simulink model "OAC_LA_Ass1_Task2_simu_R2017b"  (R2017b)
settings: Solver=VariableStepAuto  StartTime=0.0  StopTime=10.0  MaxStep=10e-3  RelTol=1e-3
undefined symbols (not defined in the file): g, l, params_L1, params_L2, params_Linfty, x0
settings Model: Creator=miko2  LastModifiedBy=miko2

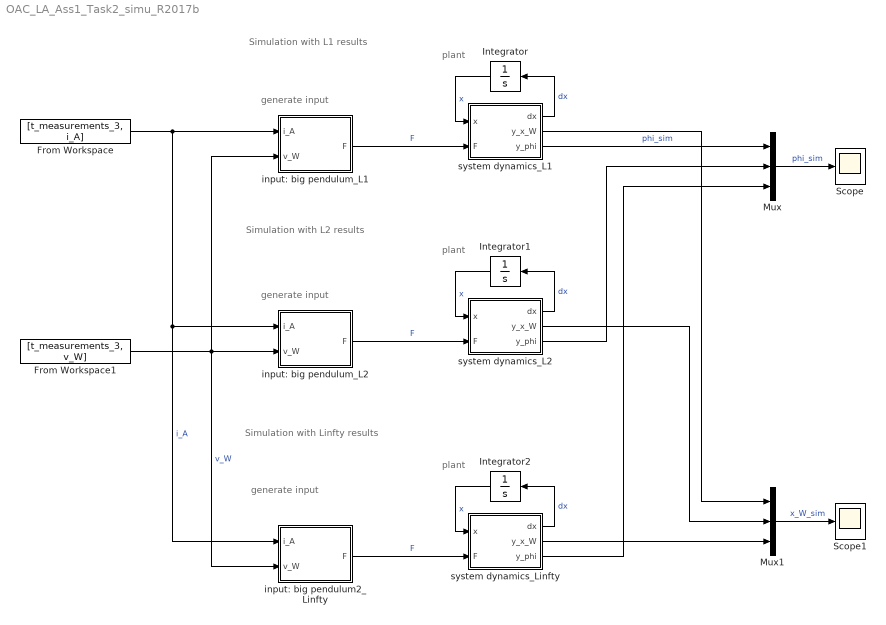
== system OAC_LA_Ass1_Task2_simu_R2017b ==
  note: Simulation with Linfty results
  note: Simulation with L2 results
  note: Simulation with L1 results
  note: generate input
  note: plant
  note: plant
  note: plant
  note: generate input
  note: generate input
  From Workspace : FromWorkspace  VariableName=[t_measurements_3, i_A]  SampleTime=0
  From Workspace1 : FromWorkspace  VariableName=[t_measurements_3, v_W]  SampleTime=0
  Integrator : Integrator  InitialCondition=x0
  Integrator1 : Integrator  InitialCondition=x0
  Integrator2 : Integrator  InitialCondition=x0
  Mux : Mux  Inputs=3
  Mux1 : Mux  Inputs=3
  Scope : Scope
  Scope1 : Scope
  input: big pendulum2_Linfty : MATLAB Function  TreatAsAtomicUnit=on
  input: big pendulum_L1 : MATLAB Function  TreatAsAtomicUnit=on
  input: big pendulum_L2 : MATLAB Function  TreatAsAtomicUnit=on
  system dynamics_L1 : MATLAB Function  TreatAsAtomicUnit=on
  system dynamics_L2 : MATLAB Function  TreatAsAtomicUnit=on
  system dynamics_Linfty : MATLAB Function  TreatAsAtomicUnit=on
  wires:
  system dynamics_L1/3(y_phi) -> Mux/1  "phi_sim"
  Integrator/1 -> system dynamics_L1/1(x)  "x"
  input: big pendulum_L1/1(F) -> system dynamics_L1/2(F)  "F"
  From Workspace/1 -> input: big pendulum_L1/1(i_A), input: big pendulum_L2/1(i_A), input: big pendulum2_Linfty/1(i_A)  "i_A"
  From Workspace1/1 -> input: big pendulum_L2/2(v_W), input: big pendulum_L1/2(v_W), input: big pendulum2_Linfty/2(v_W)  "v_W"
  system dynamics_L1/1(dx) -> Integrator/1  "dx"
  Integrator1/1 -> system dynamics_L2/1(x)  "x"
  system dynamics_L2/1(dx) -> Integrator1/1  "dx"
  system dynamics_L2/3(y_phi) -> Mux/2
  Integrator2/1 -> system dynamics_Linfty/1(x)  "x"
  system dynamics_Linfty/1(dx) -> Integrator2/1  "dx"
  system dynamics_Linfty/3(y_phi) -> Mux/3
  input: big pendulum_L2/1(F) -> system dynamics_L2/2(F)  "F"
  input: big pendulum2_Linfty/1(F) -> system dynamics_Linfty/2(F)  "F"
  Mux/1 -> Scope/1  "phi_sim"
  system dynamics_L1/2(y_x_W) -> Mux1/1
  system dynamics_L2/2(y_x_W) -> Mux1/2
  system dynamics_Linfty/2(y_x_W) -> Mux1/3
  Mux1/1 -> Scope1/1  "x_W_sim"

== matlab function OAC_LA_Ass1_Task2_simu_R2017b/input: big pendulum_L1 ==
  data: i_A input; v_W input; F output; params_L1 parameter
function F = fcn(i_A, v_W, params_L1)
    
    V = params_L1(3);
    k1 = params_L1(4);

    F = V*i_A - k1*v_W;

end

== matlab function OAC_LA_Ass1_Task2_simu_R2017b/system dynamics_L1 ==
  data: dx output; x input; y_x_W output; F input; y_phi output; params_L1 parameter; l parameter; g parameter
function [dx, y_x_W, y_phi] = fcn(x,F,params_L1,l,g)

    ms = params_L1(1);
    mw = params_L1(2);
    
    x_W = x(1);
    phi = x(2);
    v_W = x(3);
    omega = x(4);

    dx_W = v_W;
    dphi = omega;
    dv_W = 1/( mw + ms*(1-(cos(phi))^2) ) * ( F + ms*l*omega^2*sin(phi) ...
        - ms*g*sin(phi)*cos(phi) );
    domega = 1/( l * ( 1 - ms/(mw+ms)*(cos(phi))^2 ) ) * ( g*sin(phi) - ...
        cos(phi)/(ms+mw)*F - ms/(mw+ms)*l*omega^2*sin(phi)*cos(phi) );
    
    dx = [dx_W; dphi; dv_W; domega]; 
          
    y_x_W = x_W;
    y_phi = phi;

end

== matlab function OAC_LA_Ass1_Task2_simu_R2017b/system dynamics_L2 ==
  data: dx output; x input; y_x_W output; F input; y_phi output; params_L2 parameter; l parameter; g parameter
function [dx, y_x_W, y_phi] = fcn(x,F,params_L2,l,g)

    ms = params_L2(1);
    mw = params_L2(2);
    
    x_W = x(1);
    phi = x(2);
    v_W = x(3);
    omega = x(4);

    dx_W = v_W;
    dphi = omega;
    dv_W = 1/( mw + ms*(1-(cos(phi))^2) ) * ( F + ms*l*omega^2*sin(phi) ...
        - ms*g*sin(phi)*cos(phi) );
    domega = 1/( l * ( 1 - ms/(mw+ms)*(cos(phi))^2 ) ) * ( g*sin(phi) - ...
        cos(phi)/(ms+mw)*F - ms/(mw+ms)*l*omega^2*sin(phi)*cos(phi) );
    
    dx = [dx_W; dphi; dv_W; domega]; 
          
    y_x_W = x_W;
    y_phi = phi;

end

== matlab function OAC_LA_Ass1_Task2_simu_R2017b/system dynamics_Linfty ==
  data: dx output; x input; y_x_W output; F input; y_phi output; params_Linfty parameter; l parameter; g parameter
function [dx, y_x_W, y_phi] = fcn(x,F,params_Linfty,l,g)

    ms = params_Linfty(1);
    mw = params_Linfty(2);
    
    x_W = x(1);
    phi = x(2);
    v_W = x(3);
    omega = x(4);

    dx_W = v_W;
    dphi = omega;
    dv_W = 1/( mw + ms*(1-(cos(phi))^2) ) * ( F + ms*l*omega^2*sin(phi) ...
        - ms*g*sin(phi)*cos(phi) );
    domega = 1/( l * ( 1 - ms/(mw+ms)*(cos(phi))^2 ) ) * ( g*sin(phi) - ...
        cos(phi)/(ms+mw)*F - ms/(mw+ms)*l*omega^2*sin(phi)*cos(phi) );
    
    dx = [dx_W; dphi; dv_W; domega]; 
          
    y_x_W = x_W;
    y_phi = phi;

end

== matlab function OAC_LA_Ass1_Task2_simu_R2017b/input: big pendulum_L2 ==
  data: i_A input; v_W input; F output; params_L2 parameter
function F = fcn(i_A, v_W, params_L2)
    
    V = params_L2(3);
    k1 = params_L2(4);

    F = V*i_A - k1*v_W;

end

== matlab function OAC_LA_Ass1_Task2_simu_R2017b/input: big pendulum2_Linfty ==
  data: i_A input; v_W input; F output; params_Linfty parameter
function F = fcn(i_A, v_W, params_Linfty)
    
    V = params_Linfty(3);
    k1 = params_Linfty(4);

    F = V*i_A - k1*v_W;

end
